simulink model "week1_prob7"  (R2020b)
settings: Solver=VariableStepAuto  StartTime=0.0  StopTime=10.0  RelTol=1e-3
settings Model: Creator=lalit  LastModifiedBy=lalit

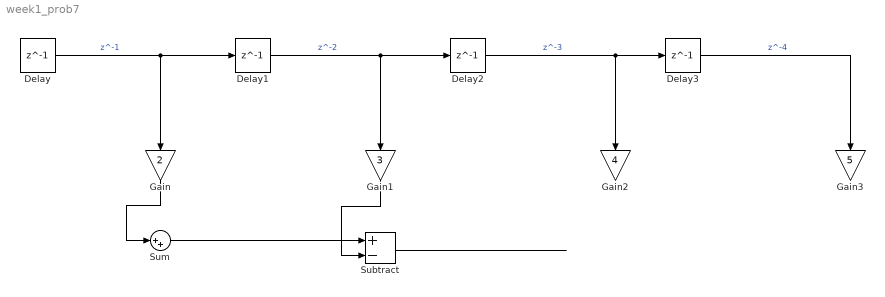
== system week1_prob7 ==
  Delay{,1..3} (4 alike) : Delay  DelayLength=1
  Gain : Gain  Gain=2
  Gain1 : Gain  Gain=3
  Gain2 : Gain  Gain=4
  Gain3 : Gain  Gain=5
  Subtract : Sum  Inputs=+-
  Sum : Sum  Inputs=|++
  wires:
  Delay/1 -> Delay1/1, Gain/1  "z^-1"
  Delay1/1 -> Gain1/1, Delay2/1  "z^-2"
  Delay2/1 -> Delay3/1, Gain2/1  "z^-3"
  ? -> Sum/2, Delay/1
  Delay3/1 -> Gain3/1  "z^-4"
  Gain/1 -> Sum/1
  Sum/1 -> Subtract/1
  Gain1/1 -> Subtract/2
  Subtract/1 -> ?
